simulink model "perrottaC1"  (R2020b)
settings: Solver=FixedStepDiscrete  StartTime=0.0  StopTime=200  FixedStep=Ts  RelTol=1e-3
model workspace (MAT data in the model file):
  Ts = 0.002
  acoeff = 0.95
  amax = 0.1
  jcoeff = 0.1
  jmax = 1
  pf = 160
  reference_command = [0 0.002 0.004 0.006 0.008 0.01 0.012 0.014 0.016 0.018 0.02 0.022 ... (200002 elements, 100001x2)]
  v = 50
  vmax = 1.5
libraries: simulink x3
(part 2 of 2)

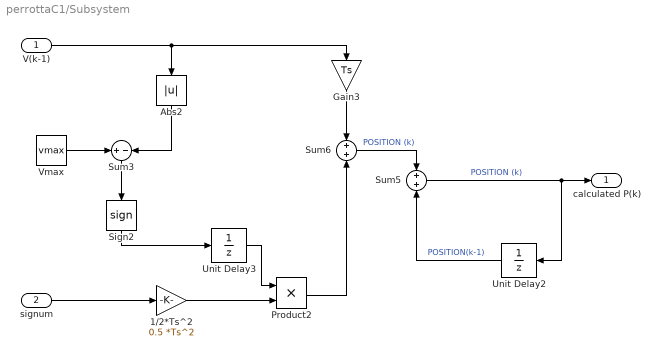
== system perrottaC1/Subsystem ==
  V(k-1) : Inport
  signum : Inport  Port=2
  1/2*Ts^2 : Gain  Gain=0.5 *Ts^2
  Abs2 : Abs
  Gain3 : Gain  Gain=Ts
  Product2 : Product
  Sign2 : Signum
  Sum3 : Sum  Inputs=+-
  Sum5 : Sum
  Sum6 : Sum
  Unit Delay2 : UnitDelay  SampleTime=-1  HasFrameUpgradeWarning=on
  Unit Delay3 : UnitDelay  SampleTime=-1  HasFrameUpgradeWarning=on
  Vmax : Constant  Value=vmax
  calculated P(k) : Outport
  wires:
  V(k-1)/1 -> Gain3/1, Abs2/1
  signum/1 -> 1/2*Ts^2/1
  Gain3/1 -> Sum6/1
  Sign2/1 -> Unit Delay3/1
  Unit Delay2/1 -> Sum5/2  "POSITION(k-1)"
  Unit Delay3/1 -> Product2/1
  1/2*Ts^2/1 -> Product2/2
  Sum3/1 -> Sign2/1
  Sum5/1 -> Unit Delay2/1, calculated P(k)/1  "POSITION (k)"
  Product2/1 -> Sum6/2
  Sum6/1 -> Sum5/1  "POSITION (k)"
  Vmax/1 -> Sum3/1
  Abs2/1 -> Sum3/2
